simulink model "psb3phPWM"  (Simulink 6.0)
settings: Solver=FixedStepDiscrete  SolverMode=SingleTasking  StartTime=0.0  StopTime=0.1  FixedStep=Ts  RelTol=1e-3
PreLoadFcn:
  | assignin('base','Ts',[1/60/3240])
InitFcn:
  | powericon('psbinitsys',bdroot);
undefined symbols (not defined in the file or in its folder): D1, Delta, Ts
libraries: powerlib2 x18, powerlib_extras x2
settings Model: Creator=patrice  LastModifiedBy=batserve  ExtModeTrigMode=oneshot  ExtModeArmWhenConnect=off  ExtModeAutoUpdateStatusClock=off
settings DataIOCC: LimitDataPoints=off  SignalLoggingName=sigsOut
settings OptimizationCC: BlockReduction=off  BooleanDataType=off
settings DebuggingCC: CheckExecutionContextPreStartOutputMsg=on  CheckExecutionContextRuntimeOutputMsg=on  SolverPrmCheckMsg=none
settings HardwareCC: TargetUnknown=on
settings RTWCC: TemplateMakefile=grt_unix.tmf

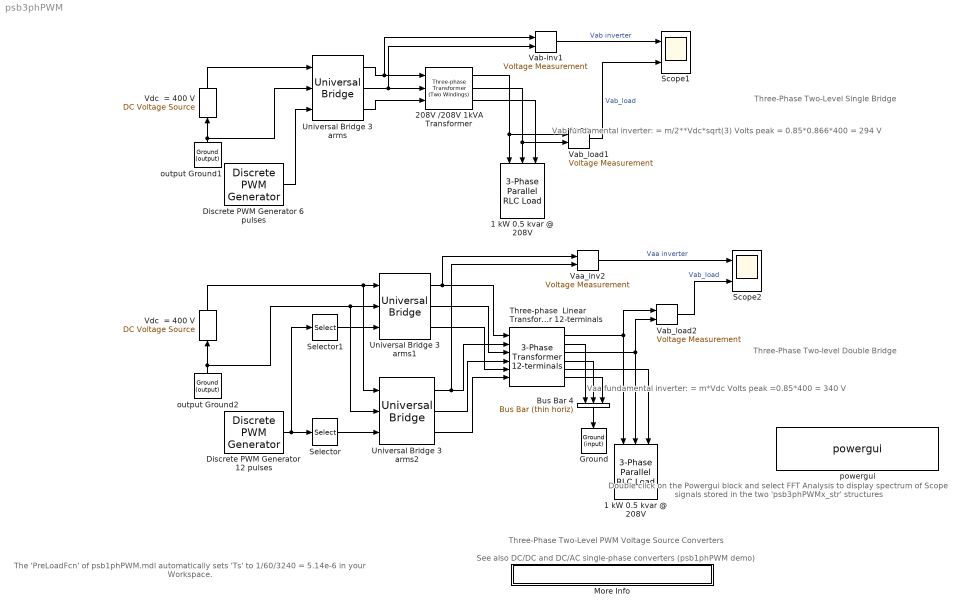
== system psb3phPWM ==
  note: Vaa fundamental inverter:
      | = m*Vdc Volts peak
      | =0.85*400
      | = 340 V
  note: Three-Phase Two-Level PWM Voltage Source Converters
  note: See also DC/DC and DC/AC single-phase converters (psb1phPWM demo)
  note: The 'PreLoadFcn' of psb1phPWM.mdl automatically
      | sets 'Ts' to 1/60/3240 = 5.14e-6 in your Workspace.
  note: Vab fundamental inverter:
      | = m/2**Vdc*sqrt(3) Volts peak
      | = 0.85*0.866*400
      | = 294 V
  note: Three-Phase Two-Level Single Bridge
  note: Three-Phase Two-level Double Bridge
  note: Double click on the Powergui block and
      | select FFT Analysis to display spectrum
      | of Scope  signals stored in the two
      | 'psb3phPWMx_str' structures
  1 kW 0.5 kvar @ 208V : powerlib2/Elements/3-Phase Parallel RLC Load  Orientation=down  Vpp=208  fn=60  P3=1000  QL3=0  QC3=500
  "1 kW 0.5 kvar @ 208V " : powerlib2/Elements/3-Phase Parallel RLC Load  Orientation=down  Vpp=208  fn=60  P3=1000  QL3=0  QC3=500
  208V /208V 1kVA Transformer : powerlib2/Elements/Three-phase Transformer (Two Windings)  Tag=PoWeRsYsTeMbLoCk  nominal=[ 1000 , 60 ]  type1=Delta (D1)  params1=[ 208 , 0.002 , 0.04 ]  type2=Yg  params2=[ 208 , 0.002 , 0.04 ]  ynsat=off  rmag=200  lm=200  sat="[ 0,0  ;  0.005,1.2  ;  1.0,1.4 ]"  hyst=off  matfile='hysteresis'  sif=off  phi0=[ 0.8 , -0.8 , 0.7 ]  initialslopes=[+1 +1 +1]  mesure=None  PSBOutputType=1111
  Bus Bar 4 : powerlib2/Connectors/Bus Bar (thin horiz)  Tag=PoWeRsYsTeMbLoCk  Orientation=down  input=3  output=1  PSBOutputType=111111111111111111111111111111111111111111111111111111111111111111111111111111111111
  Discrete PWM Generator 12 pulses : powerlib_extras/Discrete  Control Blocks/Discrete PWM Generator  GeneratorMode="Double 3-arm  bridges (12 pulses)"  Fc=1080  Ts=Ts  Internal=on  mIndex=0.85  Freq=60  Phase=0
  Discrete PWM Generator 6 pulses : powerlib_extras/Discrete  Control Blocks/Discrete PWM Generator  GeneratorMode="3-arm  bridge (6 pulses)"  Fc=1080  Ts=Ts  Internal=on  mIndex=0.85  Freq=60  Phase=0
  Ground : powerlib2/Connectors/Ground (input)  Tag=PoWeRsYsTeMbLoCk  Orientation=down
  More Info : Subsystem
      mask Display: disp('? : Double-click here for more info')
  Scope1 : Scope  NumInputPorts=2
      settings: TimeRange=0.1  YMin=-500~-400  YMax=500~500  SaveName=psb3phPWM1_str  MaxDataPoints=500000
  Scope2 : Scope  NumInputPorts=2
      settings: TimeRange=0.1  YMin=-500~-300  YMax=500~400  SaveName=psb3phPWM2_str  MaxDataPoints=500000
  Selector : Selector  Elements=7:12  InputPortWidth=12
  Selector1 : Selector  Elements=1:6  InputPortWidth=12
  "Three-phase  Linear Transformer 12-terminals " : powerlib2/Elements/3-Phase Transformer 12-terminals  pf=[ 1000 60 ]  urx1="[ 240  0.002  0.04 ]"  urx2=[ 208/sqrt(3) 0.002 0.04]  rxm=[ 200 200 ]
  Universal Bridge 3 arms : powerlib2/Power Electronics/Universal Bridge  Tag=PoWeRsYsTeMbLoCk  arms=3  confi=ABC as output terminals  injcc=10000  cf=inf  device=IGBT / Diodes  Ron=1e-4  Lon=0  VFs="[  1  1  ]"  Vf=.8  gtoparameters=[ 10e-6 , 20e-6 ]  igbtparameters=[ 1e-6 , 2e-6 ]  mesure=None  PSBOutputType=111
  Universal Bridge 3 arms1 : powerlib2/Power Electronics/Universal Bridge  Tag=PoWeRsYsTeMbLoCk  arms=3  confi=ABC as output terminals  injcc=10000  cf=inf  device=IGBT / Diodes  Ron=1e-4  Lon=0  VFs="[  1  1  ]"  Vf=.8  gtoparameters=[ 10e-6 , 20e-6 ]  igbtparameters=[ 1e-6 , 2e-6 ]  mesure=None  PSBOutputType=111
  Universal Bridge 3 arms2 : powerlib2/Power Electronics/Universal Bridge  Tag=PoWeRsYsTeMbLoCk  arms=3  confi=ABC as output terminals  injcc=10000  cf=inf  device=IGBT / Diodes  Ron=1e-4  Lon=0  VFs="[  1  1  ]"  Vf=.8  gtoparameters=[ 10e-6 , 20e-6 ]  igbtparameters=[ 1e-6 , 2e-6 ]  mesure=None  PSBOutputType=111
  Vaa_inv2 : powerlib2/Measurements/Voltage Measurement  Tag=PoWeRsYsTeMmEaSuReMeNt  PhasorSimulation=off  OutputType=Magnitude  PSBOutputType=0  PSBequivalent=0
  Vab-inv1 : powerlib2/Measurements/Voltage Measurement  Tag=PoWeRsYsTeMmEaSuReMeNt  PhasorSimulation=off  OutputType=Magnitude  PSBOutputType=0  PSBequivalent=0
  Vab_load1 : powerlib2/Measurements/Voltage Measurement  Tag=PoWeRsYsTeMmEaSuReMeNt  PhasorSimulation=off  OutputType=Magnitude  PSBOutputType=0  PSBequivalent=0
  Vab_load2 : powerlib2/Measurements/Voltage Measurement  Tag=PoWeRsYsTeMmEaSuReMeNt  PhasorSimulation=off  OutputType=Magnitude  PSBOutputType=0  PSBequivalent=0
  Vdc  = 400 V : powerlib2/Electrical Sources/DC Voltage Source  Tag=PoWeRsYsTeMbLoCk  Orientation=up  V=400  mesure=None  PSBOutputType=1
  "Vdc  = 400 V " : powerlib2/Electrical Sources/DC Voltage Source  Tag=PoWeRsYsTeMbLoCk  Orientation=up  V=400  mesure=None  PSBOutputType=1
  output Ground1 : powerlib2/Connectors/Ground (output)  Tag=PoWeRsYsTeMbLoCk  Orientation=up  PSBOutputType=1
  output Ground2 : powerlib2/Connectors/Ground (output)  Tag=PoWeRsYsTeMbLoCk  Orientation=up  PSBOutputType=1
  powergui : powerlib2/powergui  Frange=[0:2:500]  Ylog=off  Xlog=off  save=off  variable=ZData  structure=psb3phPWM1_str  ZoomFFT=on  StartTime=0.1-2/60  cycles=2  DisplayStyle=off  fundamental=60  FreqAxis=off  MaxFrequency=5000  frequencyindice=1  frequencyindicesteady=1  RmsSteady=1  display=off  Ts=Ts  methode=off  frequency=60  echomessages=off
  wires:
  Discrete PWM Generator 6 pulses/1 -> Universal Bridge 3 arms/3
  Universal Bridge 3 arms/1 -> Vab-inv1/1, 208V /208V 1kVA Transformer/1
  Universal Bridge 3 arms/2 -> Vab-inv1/2, 208V /208V 1kVA Transformer/2
  Universal Bridge 3 arms/3 -> 208V /208V 1kVA Transformer/3
  Vab_load1/1 -> Scope1/2  "Vab_load"
  208V /208V 1kVA Transformer/3 -> 1 kW 0.5 kvar @ 208V/3
  208V /208V 1kVA Transformer/1 -> 1 kW 0.5 kvar @ 208V/1, Vab_load1/1
  208V /208V 1kVA Transformer/2 -> 1 kW 0.5 kvar @ 208V/2, Vab_load1/2
  Vab-inv1/1 -> Scope1/1  "Vab inverter"
  Discrete PWM Generator 12 pulses/1 -> Selector/1, Selector1/1
  Selector1/1 -> Universal Bridge 3 arms1/3
  Selector/1 -> Universal Bridge 3 arms2/3
  "Vdc  = 400 V "/1 -> Universal Bridge 3 arms1/1, Universal Bridge 3 arms2/1
  Universal Bridge 3 arms1/2 -> "Three-phase  Linear Transformer 12-terminals "/3
  Universal Bridge 3 arms2/2 -> "Three-phase  Linear Transformer 12-terminals "/4
  Universal Bridge 3 arms2/3 -> "Three-phase  Linear Transformer 12-terminals "/6
  Universal Bridge 3 arms1/3 -> "Three-phase  Linear Transformer 12-terminals "/5
  Universal Bridge 3 arms1/1 -> "Three-phase  Linear Transformer 12-terminals "/1, Vaa_inv2/1
  Universal Bridge 3 arms2/1 -> "Three-phase  Linear Transformer 12-terminals "/2, Vaa_inv2/2
  "Three-phase  Linear Transformer 12-terminals "/1 -> "1 kW 0.5 kvar @ 208V "/1, Vab_load2/1
  output Ground2/1 -> "Vdc  = 400 V "/1, Universal Bridge 3 arms1/2, Universal Bridge 3 arms2/2
  Vaa_inv2/1 -> Scope2/1  "Vaa inverter"
  Vab_load2/1 -> Scope2/2  "Vab_load"
  Vdc  = 400 V/1 -> Universal Bridge 3 arms/1
  output Ground1/1 -> Vdc  = 400 V/1, Universal Bridge 3 arms/2
  "Three-phase  Linear Transformer 12-terminals "/2 -> Bus Bar 4/1
  Bus Bar 4/1 -> Ground/1
  "Three-phase  Linear Transformer 12-terminals "/4 -> Bus Bar 4/2
  "Three-phase  Linear Transformer 12-terminals "/6 -> Bus Bar 4/3
  "Three-phase  Linear Transformer 12-terminals "/3 -> "1 kW 0.5 kvar @ 208V "/2, Vab_load2/2
  "Three-phase  Linear Transformer 12-terminals "/5 -> "1 kW 0.5 kvar @ 208V "/3

== system psb3phPWM/More Info ==
  note: G. Sybille and P. Giroux (Hydro-Quebec)
  note: Demonstration
  note: Circuit Description
  note: This demonstration illustrates use of the Universal Bridge and
      | Discrete PWM Pulse Generator blocks. It also demonstrates
      | harmonic analysis of PWM waveforms using the Powergui/FFT tool.
  note: The system consists of two independant circuits illustrating two three-phase two-level PWM voltage source inverters.
      | Each  inverter feeds an AC load (1 kW, 500 var 60Hz @ 208V rms) through a three-phase transformer.
      | Both converters are controlled in open loop with the Discrete PWM Generator block available in the Extras/Discrete Control Blocks library.
      | The two circuits use the same DC voltage (Vdc = 400V), carrier frequency (1080 Hz), modulation index (m = 0.85) and generated frequency (f = 60 Hz).
      | Harmonic filtering is performed by the transformer leakage inductance (8%) and load capacitance (500 var).
      | The two circuits are:
      |
      | 1. Three-phase,  two-level converter (one three-arm bridge; six-switches)
      | 2. Three-phase,  two-level converter (two three-arm bridge; twelve-switches in H configuration)
      |
      | In order to allow further signal processing, signals displayed on the two Scope blocks  (sampled at simulation sampling rate of 3240 samples/ cycle)
      | are stored in two  variables named 'psb3phPWM1_str' and 'psb3phPWM2_str'  (structures with time) .
  note: Run the simulation and observe the following two waveforms on the Scope blocks:
      | Voltage generated by the PWM inverter (trace 1), load voltage (trace 2)
      |
      | Once the  simulation is completed, open the Powergui and select  'FFT Analysis' to display the 0-5000 Hz frequency spectrum of signals saved
      | in the two 'psb3phPWMx_str' structures. The FFT will be performed on  a 2-cycle window starting at t = 0.1 - 2/60 (last 2 cycles of recording).
      | For each circuit selelect Input labeled 'Vaa inverter'  or 'Vab inveter'. Click on Display and observe the frequency spectrum of last 2 cycles.
      |
      | The fundamental component of  V inverter is displayed above the spectrum window.
      | Compare the magnitude of the fundamental of the inverter voltage with the theoretical values given in the  circuit.
      |
      | Compare also the harmonic contents in the inverter voltage for the two-switch and four-switch DC/AC inverters.
      | For the six-switch inverter,  the first harmonics  occur around the carrier frequency (1080 Hz +- k*60Hz)
      | whereas for the twelve-switch inverter harmonics are lower and appear at double of carrier frequency
      | As a result, the load voltage is "cleaner" for the twelve-switch inverter.
      | If you now perform a FFT on the signal Vab_load you will notice that the THD  is 4,1% for the six-switch inverter as compared to
      | only 1.7% for the twelve-switch inverter.
